simulink model "Manoel_03"  (R2018a)
settings: Solver=VariableStepAuto  StartTime=0.0  StopTime=10.0  RelTol=1e-3
values from neighbouring files (symbols this model uses):
  atraso = stt    [manoel_outubro2.m]    (also in naao_roda.m = infor.SettlingTime; pre6_teste.m = infor.SettlingTime; pre_lab3.m = infor.SettlingTime; pre_lab3_lab.m = infor.SettlingTime)
  b0 = 18    [naao_roda.m]    (also in pre6_teste.m; pre_lab3.m; pre_lab3_2.m; pre_lab3_lab.m)
  ganho = 0.01027*infor.SettlingMax    [manoel_outubro2.m]    (also in naao_roda.m; pre6_teste.m; pre_lab3.m; pre_lab3_lab.m)
  Kpf = 1.0436    [pre_lab3.m]    (also in pre_lab3_lab.m; pre_lab4.m; pre_pedro.m = 1/dcgain(EE))
  q0c = 0.4    [naao_roda.m]
  q1c = 0.977    [naao_roda.m]
  R0 = round(r0,1)    [naao_roda.m]    (also in pre6_teste.m; pre_lab3.m; pre_lab3_lab.m; pre_lab4.m)
  T0 = round(t0,3)    [naao_roda.m]    (also in pre6_teste.m = 0.063; pre_lab3.m; pre_lab3_2.m = 0.0640576; pre_lab3_lab.m)
  Umax = 10    [naao_roda.m]    (also in pre6_teste.m; pre_lab3.m; pre_lab3_lab.m; pre_lab4.m)
undefined symbols (not defined in the file or in its folder): q0p
settings Model: Creator=joaovitor  LastModifiedBy=joaovitor

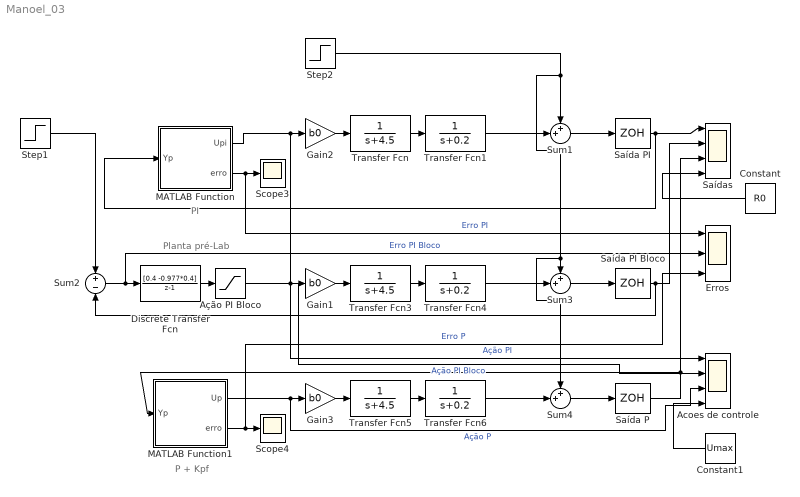
== system Manoel_03 ==
  note: Planta pré-Lab
  note: PI
  note: P + Kpf
  Acoes de controle : Scope  NumInputPorts=4
  Ação PI Bloco : Saturate  UpperLimit=10  LowerLimit=-10
  Constant : Constant  Value=R0
  Constant1 : Constant  Value=Umax
  Discrete Transfer Fcn : DiscreteTransferFcn  Numerator=[0.4 -0.977*0.4]  Denominator=[1 -1]  SampleTime=T0
  Erros : Scope  NumInputPorts=3
  Gain1 : Gain  Gain=b0
  Gain2 : Gain  Gain=b0
  Gain3 : Gain  Gain=b0
  MATLAB Function : MATLAB Function  TreatAsAtomicUnit=on
  MATLAB Function1 : MATLAB Function  TreatAsAtomicUnit=on
  Saída P : ZeroOrderHold  SampleTime=T0
  Saída PI : ZeroOrderHold  SampleTime=T0
  Saída PI Bloco : ZeroOrderHold  SampleTime=T0
  Saídas : Scope  NumInputPorts=4
  Scope3 : Scope
  Scope4 : Scope
  Step1 : Step  Time=0  After=R0  SampleTime=0
  Step2 : Step  Time=3*atraso  After=25*ganho  SampleTime=0
  Sum1 : Sum  Inputs=++|
  Sum2 : Sum  Inputs=+|-
  Sum3 : Sum  Inputs=++|
  Sum4 : Sum  Inputs=++|
  Transfer Fcn : TransferFcn  Denominator=[1 4.5]
  Transfer Fcn1 : TransferFcn  Denominator=[1 0.2]
  Transfer Fcn3 : TransferFcn  Denominator=[1 4.5]
  Transfer Fcn4 : TransferFcn  Denominator=[1 0.2]
  Transfer Fcn5 : TransferFcn  Denominator=[1 4.5]
  Transfer Fcn6 : TransferFcn  Denominator=[1 0.2]
  wires:
  MATLAB Function/1(Upi) -> Acoes de controle/1, Gain2/1  "Ação PI"
  Gain2/1 -> Transfer Fcn/1
  Transfer Fcn/1 -> Transfer Fcn1/1
  Transfer Fcn1/1 -> Sum1/2
  Sum1/1 -> Saída PI/1
  Step2/1 -> Sum4/1, Sum3/1, Sum1/1
  Step1/1 -> Sum2/1
  Saída PI/1 -> Saídas/1, MATLAB Function/1(Yp)
  MATLAB Function/2(erro) -> Erros/1, Scope3/1  "Erro PI"
  Discrete Transfer Fcn/1 -> Ação PI Bloco/1
  Transfer Fcn3/1 -> Transfer Fcn4/1
  Gain1/1 -> Transfer Fcn3/1
  Ação PI Bloco/1 -> Acoes de controle/2, Gain1/1  "Ação PI Bloco"
  Transfer Fcn4/1 -> Sum3/2
  Sum3/1 -> Saída PI Bloco/1
  Saída PI Bloco/1 -> Saídas/2, Sum2/2
  Transfer Fcn5/1 -> Transfer Fcn6/1
  Gain3/1 -> Transfer Fcn5/1
  Transfer Fcn6/1 -> Sum4/2
  Sum4/1 -> Saída P/1
  Saída P/1 -> Saídas/3, MATLAB Function1/1(Yp)
  MATLAB Function1/1(Up) -> Acoes de controle/3, Gain3/1  "Ação P"
  MATLAB Function1/2(erro) -> Erros/3, Scope4/1  "Erro P"
  Sum2/1 -> Erros/2, Discrete Transfer Fcn/1  "Erro PI Bloco"
  Constant/1 -> Saídas/4
  Constant1/1 -> Acoes de controle/4

== matlab function Manoel_03/MATLAB Function1 ==
  data: Up output; Yp input; erro output; R0 parameter; q0p parameter; Umax parameter; Kpf parameter
function [Up,erro] = fcn(Yp, R0, q0p, Umax, Kpf)    

erro=Kpf*R0-Yp
Up=q0p*erro;

if(abs(Up)>Umax)
    Up=Umax*sign(Up)

end

== matlab function Manoel_03/MATLAB Function ==
  data: Yp input; Upi output; erro output; R0 parameter; q0c parameter; Umax parameter; Kpf parameter; q1c parameter
function [Upi,erro] = fcn(Yp, R0, q0c, Umax, Kpf, q1c)    
  
persistent u0; 
persistent e0;

if isempty(u0)
    u0=0;
    e0=0;
end

erro=R0-Yp
Upi=u0+q0c*erro-q1c*q0c*e0;

u0=Upi;
e0=erro;

if(abs(Upi)>Umax)
    Upi=Umax*sign(Upi)

end
